simulink library "Collector_1xN"  (Simulink 8.2)
settings: Solver=ode45  StartTime=0.0  StopTime=10.0  RelTol=1e-3
libraries: carnot x5
settings Model: Creator=lena.frank  LastModifiedBy=drhf

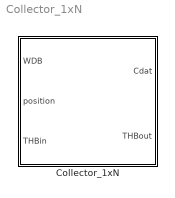
== system Collector_1xN ==
  Collector_1xN : Subsystem  mask(collector){acol=2.3, len=2, eta0=0.8, u1=3.5, u2=0.02, u3=0, uwind=0, c_col=1e4, lin=10, qua=10, tini=20, nodes=5}
      mask prompts: acol "collector surface (aperture) in [m²]"; len "length between inlet and outlet [m]"; eta0 "optical efficiency [-]"; u1 "linear heat loss coefficient [W/(m²*K)]"; u2 "quadratic heat loss coefficient [W/(m*K)²]"; u3 "radiative loss coefficient [W/(m²*K)]"; uwind "wind dependent heat loss [W/(m²*K*m/s)]"; c_col "effective heat capacity of collector [J/(m²*K)]"; lin "linear pressure drop Pa/(kg/s)"; qua "quadratic  pressure drop Pa/(kg/s)²"; tini "initial temperature [degree Celsius]"; nodes "number of nodes"
      mask help:
      | Model for tested collectors. Enter test results in this mask.
      | Look under mask to change the incidence angle modifier, the pressure drop and the radiation calculation method.
      mask init:
      | acol = max(acol, 0.01);
      | eta0 = max(eta0,0);
      | c_col = max(c_col, 0.1);
      mask Help: web(fullfile(path_carnot('help'),'Collector_1xN.html'),'-helpbrowser')
      mask Display: plot(-10,0,80,78,[10 16 66 60 10],[16 10 60 66 16],[8,13],[8,13],[63,68],[63,68])

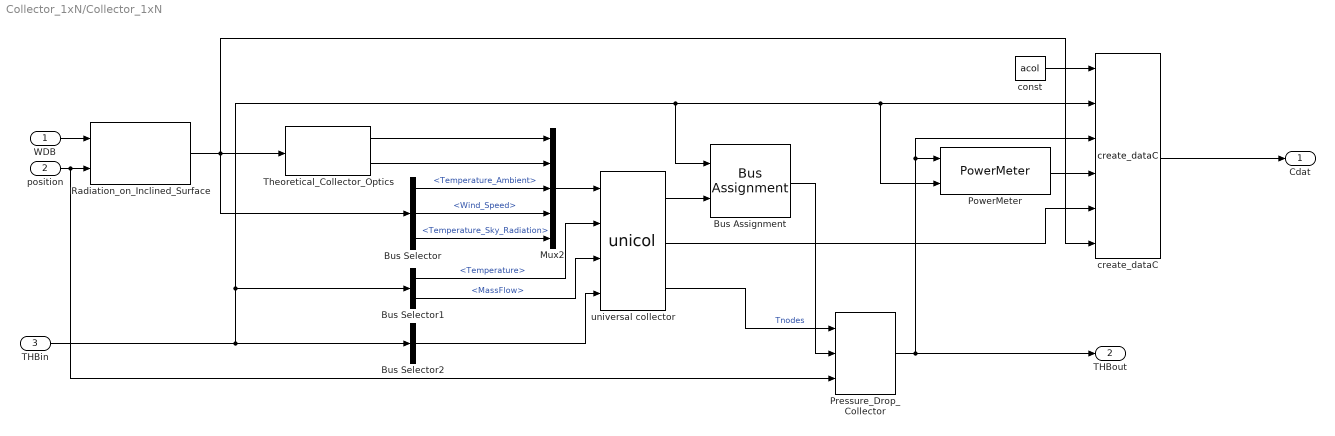
== system Collector_1xN/Collector_1xN ==
  WDB : Inport
  position : Inport  Port=2
  THBin : Inport  Port=3
  Bus Assignment : BusAssignment  AssignedSignals=Temperature
  Bus Selector : BusSelector  OutputSignals=Temperature_Ambient,Wind_Speed,Temperature_Sky_Radiation
  Bus Selector1 : BusSelector  OutputSignals=Temperature,MassFlow
  Bus Selector2 : BusSelector  OutputSignals=Pressure,FluidType,FluidMix  OutputAsBus=on
  Mux2 : Mux  Inputs=5
  PowerMeter : carnot/Control/PowerMeter
  Pressure_Drop_Collector : carnot/Basic/Pressure_Drop/Pressure_Drop_Collector  len=len  lin=lin  qua=qua
  Radiation_on_Inclined_Surface : carnot/Weather/Radiation_on_Inclined_Surface  sky=Perez 1990  reflect=0.2
  Theoretical_Collector_Optics : carnot/Source/Solar_Thermal/IncidenceAngleModifier/Theoretical_Collector_Optics  eta0=0.8  ncover=1  refin=1.525  d=0.004  ext=4
  const : Constant  Value=acol
  create_dataC : carnot/Source/Solar_Thermal/Collector_EN12975/create_dataC
  universal collector : S-Function  FunctionName=unicol  Parameters=acol, u1, u2, u3, uwind, c_col, tini, nodes  EnableBusSupport=off
  Cdat : Outport
  THBout : Outport  Port=2
  wires:
  create_dataC/1 -> Cdat/1
  const/1 -> create_dataC/1
  THBin/1 -> Bus Selector1/1, Bus Assignment/1, create_dataC/2, PowerMeter/2, Bus Selector2/1
  WDB/1 -> Radiation_on_Inclined_Surface/1
  position/1 -> Radiation_on_Inclined_Surface/2, Pressure_Drop_Collector/3
  Radiation_on_Inclined_Surface/1 -> Theoretical_Collector_Optics/1, create_dataC/6, Bus Selector/1
  universal collector/2 -> create_dataC/5
  universal collector/1 -> Bus Assignment/2
  Pressure_Drop_Collector/1 -> THBout/1, create_dataC/3, PowerMeter/1
  Bus Selector/2 -> Mux2/4  "<Wind_Speed>"
  Bus Selector/1 -> Mux2/3  "<Temperature_Ambient>"
  Theoretical_Collector_Optics/1 -> Mux2/1
  Theoretical_Collector_Optics/2 -> Mux2/2
  Bus Selector/3 -> Mux2/5  "<Temperature_Sky_Radiation>"
  Mux2/1 -> universal collector/1
  Bus Selector1/1 -> universal collector/2  "<Temperature>"
  Bus Selector1/2 -> universal collector/3  "<MassFlow>"
  Bus Selector2/1 -> universal collector/4
  PowerMeter/1 -> create_dataC/4
  universal collector/3 -> Pressure_Drop_Collector/1  "Tnodes"
  Bus Assignment/1 -> Pressure_Drop_Collector/2
